simulink model "SIL"  (R2019b)
settings: Solver=ode4  StartTime=Aircraft_Data.t_i  StopTime=Aircraft_Data.t_f  FixedStep=Aircraft_Data.dt  RelTol=1e-3
PostLoadFcn:
  | %% Adding File Path to MATLAb's Search Path
  | addpath(fileparts(which(bdroot)))
  | 
  | %% Aircraft Data
  | Data_From_Excel = readmatrix('B-747 Flight Condition 5.xlsx','Range','B2:B61');
  | Aircraft_Data = AircraftData(Data_From_Excel);
InitFcn:
  | %% Adding File Path to MATLAb's Search Path
  | addpath(fileparts(which(bdroot)))
  | 
  | %% Aircraft Data
  | Data_From_Excel = readmatrix('B-747 Flight Condition 5.xlsx','Range','B2:B61');
  | Aircraft_Data = AircraftData(Data_From_Excel);
undefined symbols (not defined in the file or in its folder): Earth, sigbuilder_block, WGS84
libraries: aerolibfltsims x2, simulink x2, aerolibtransform2 x1, simulink_extras x1
settings Model: Creator=Mahmoud A. Moustafa  LastModifiedBy=Mahmoud A. Moustafa

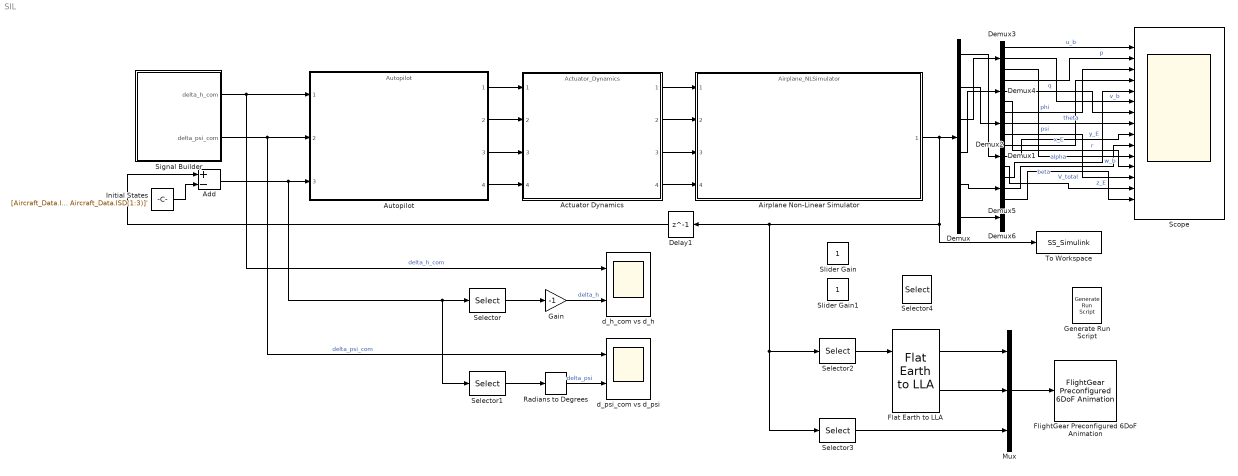
== system SIL ==
  Actuator Dynamics : ModelReference  ModelNameDialog=Actuator_Dynamics.slx  SimulationMode=Normal  ModelReferenceVersion=1.3
  Add : Sum  Inputs=+-
  Airplane Non-Linear Simulator : ModelReference  ModelNameDialog=Airplane_NLSimulator.slx  SimulationMode=Normal  ModelReferenceVersion=1.37
  Autopilot : ModelReference  ModelNameDialog=Autopilot.slx  SimulationMode=Normal  ModelReferenceVersion=1.16
  Delay1 : Delay  DelayLength=1  InitialCondition=[Aircraft_Data.ISV(10:12); Aircraft_Data.ISV(7:9); Aircraft_Data.ISV(1:3); Aircraft_Data.ISV(4:6); Aircraft_Data.ISV(13:14); Aircraft_Data.V_T0; Aircraft_Data.ISD(1:3)]'
  Demux : Demux  Outputs=6
  Demux{1..6} (6 alike) : Demux  Outputs=3
  Flat Earth to LLA : aerolibtransform2/Flat Earth to LLA  units=English  ptype=Earth (WGS84)  F=1/298.257223563  R=20925646.3255  LL0=[0 10]  psi=0
  FlightGear Preconfigured 6DoF Animation : aerolibfltsims/FlightGear Preconfigured 6DoF Animation  xFlightGearVersion=v2018.3  DestinationIpAddress=127.0.0.1  DestinationPort=5502  SampleTime=-1  packetVersion=24
  Gain : Gain  Gain=-1
  Generate Run Script : aerolibfltsims/Generate Run Script  Architecture=Default  dataFlow=Send  GeometryModelName=747-200  AirportId=KSFO  RunwayId=10L  InitialAltitude=-Aircraft_Data.ISV(12)  InitialHeading=Aircraft_Data.ISV(9)*180/pi  OffsetDistance=4.72  OffsetAzimuth=0  InstallScenery=off  DisableShaders=off  OriginAddress=127.0.0.1  DestinationPort=5502  OriginPort=5505  LocalAddress=127.0.0.1  OutputFileName=runfg.bat  FlightGearBaseDirectory=C:\Program Files\FlightGear
  Initial States : Constant  Value=[Aircraft_Data.ISV(10:12); Aircraft_Data.ISV(7:9); Aircraft_Data.ISV(1:3); Aircraft_Data.ISV(4:6); Aircraft_Data.ISV(13:14); Aircraft_Data.V_T0; Aircraft_Data.ISD(1:3)]'
  Mux : Mux  Inputs=3
  Radians to Degrees : simulink_extras/Transformations/Radians to Degrees
  Scope : Scope  NumInputPorts=15
  Selector : Selector  InputPortWidth=18  IndexOptions=Index vector (dialog)  Indices=[3]  OutputSizes=1
  Selector1 : Selector  InputPortWidth=18  IndexOptions=Index vector (dialog)  Indices=[6]  OutputSizes=1
  Selector2 : Selector  InputPortWidth=18  IndexOptions=Index vector (dialog)  Indices=[1 2 3]  OutputSizes=1
  Selector3 : Selector  InputPortWidth=18  IndexOptions=Index vector (dialog)  Indices=[4 5 6]  OutputSizes=1
  Selector4 : Selector  InputPortWidth=2  IndexOptions=Index vector (dialog)  Indices=[2 1]  OutputSizes=1
  Signal Builder : Subsystem  Tag=STV Subsys  LoadFcn=sigbuilder_block('load');  StartFcn=sigbuilder_block('start');  StopFcn=sigbuilder_block('stop');  ClipboardFcn=sigbuilder_block('clipboard');  mask(Sigbuilder block){tuvar=[0:10]}
      mask help: Simulink:masks:SigbuilderBlock_MD
      mask init:
      | if ~strcmp(get_param(bdroot(gcbh),'SimulationStatus'),'stopped') tuvar = sigbuilder_block('maskInit'); end
      settings: CopyFcn=sigbuilder_block('copy');  DeleteFcn=sigbuilder_block('delete');  ModelCloseFcn=sigbuilder_block('modelClose');  PreSaveFcn=sigbuilder_block('preSave');  PauseFcn=sigbuilder_block('pause');  ContinueFcn=sigbuilder_block('continue');  NameChangeFcn=sigbuilder_block('namechange');  OpenFcn=sigbuilder_block('open',[201 32.25 550.5 359.25 ]);  CloseFcn=sigbuilder_block('close');
      mask Display: plot(0, 0, 100, 100,[2, 2, 32, 32, 2], [68, 8, 8, 68, 68],[32, 2], [38, 38], [32, 19, 2],[53, 60, 44], [32, 17, 17, 2],[16, 16, 31, 31]);txt = getActiveGroup(gcbh);text(2, 100, txt,'verticalAlignment', 'top');
  Slider Gain : simulink/Math Operations/Slider Gain  gain=1  low=0  high=360
  Slider Gain1 : simulink/Math Operations/Slider Gain  gain=1  low=-500  high=500
  To Workspace : ToWorkspace  VariableName=SS_Simulink  SaveFormat=Timeseries  SampleTime=-1
  d_h_com vs d_h : Scope  NumInputPorts=2
  d_psi_com vs d_psi : Scope  NumInputPorts=2
  wires:
  Autopilot/1 -> Actuator Dynamics/1
  Autopilot/2 -> Actuator Dynamics/2
  Autopilot/3 -> Actuator Dynamics/3
  Autopilot/4 -> Actuator Dynamics/4
  Demux/1 -> Demux1/1
  Demux/2 -> Demux2/1
  Delay1/1 -> Add/1
  Initial States/1 -> Add/2
  Signal Builder/1(delta_h_com) -> Autopilot/1, d_h_com vs d_h/1  "delta_h_com"
  Selector/1 -> Gain/1
  Add/1 -> Autopilot/3, Selector1/1, Selector/1
  Gain/1 -> d_h_com vs d_h/2  "delta_h"
  Selector1/1 -> Radians to Degrees/1
  Signal Builder/2(delta_psi_com) -> Autopilot/2, d_psi_com vs d_psi/1  "delta_psi_com"
  Radians to Degrees/1 -> d_psi_com vs d_psi/2  "delta_psi"
  Actuator Dynamics/2 -> Airplane Non-Linear Simulator/2
  Actuator Dynamics/4 -> Airplane Non-Linear Simulator/4
  Actuator Dynamics/1 -> Airplane Non-Linear Simulator/1
  Actuator Dynamics/3 -> Airplane Non-Linear Simulator/3
  Demux/3 -> Demux3/1
  Demux/4 -> Demux4/1
  Demux/5 -> Demux5/1
  Demux/6 -> Demux6/1
  Demux3/1 -> Scope/1  "u_b"
  Demux5/3 -> Scope/15  "V_total"
  Demux3/2 -> Scope/6  "v_b"
  Demux3/3 -> Scope/11  "w_b"
  Demux4/1 -> Scope/2  "p"
  Demux2/1 -> Scope/3  "phi"
  Demux1/1 -> Scope/4  "x_E"
  Demux5/1 -> Scope/5  "alpha"
  Demux4/2 -> Scope/7  "q"
  Demux2/2 -> Scope/8  "theta"
  Demux1/2 -> Scope/9  "y_E"
  Demux5/2 -> Scope/10  "beta"
  Demux4/3 -> Scope/12  "r"
  Demux2/3 -> Scope/13  "psi"
  Demux1/3 -> Scope/14  "z_E"
  Flat Earth to LLA/2 -> Mux/2
  Selector3/1 -> Mux/3
  Flat Earth to LLA/1 -> Mux/1
  Mux/1 -> FlightGear Preconfigured 6DoF Animation/1
  Selector2/1 -> Flat Earth to LLA/1
  Airplane Non-Linear Simulator/1 -> To Workspace/1, Selector3/1, Selector2/1, Delay1/1, Demux/1

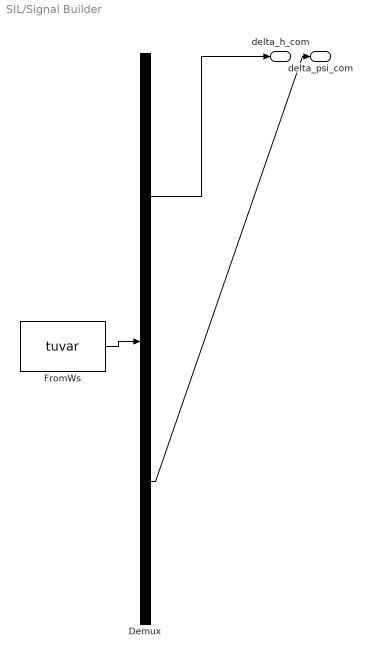
== system SIL/Signal Builder ==
  Demux : Demux  Tag=STV Demux  Outputs=2
  FromWs : FromWorkspace  Tag=STV FromWs  VariableName=tuvar  SampleTime=0
      SigBuilderData=|
      | common.afterFinalStr = 'Extrapolate'
      | common.sampleTime = 0
      | dataSet.timeRange = [0 1800]
      | dataSet.name = 'Group 1'
      | sbobj.Groups.Name = 'Group 1'
      | sbobj.Groups.Signals(1).Name = 'delta_h_com'
      | sbobj.Groups.Signals(1).XData = [0 600 1080 1080 1200 1800]
      | sbobj.Groups.Signals(1).YData = [0 10000 10000 10100 10100 0]
      | sbobj.Groups.Signals(2).Name = 'delta_psi_com'
      | sbobj.Groups.Signals(2).XData = [0 720 720 1080 1080 1800]
      | sbobj.Groups.Signals(2).YData = [0 0 360 360 390 390]
      | sbobj.Groups.TimeRange = [0 1800]
  delta_h_com : Outport  Tag=STV Outport
  delta_psi_com : Outport  Tag=STV Outport  Port=2
  wires:
  Demux/1 -> delta_h_com/1
  FromWs/1 -> Demux/1
  Demux/2 -> delta_psi_com/1
